simulink model "APFI_MI"  (R2025a)
settings: Solver=VariableStepAuto  StartTime=0.0  StopTime=1  RelTol=1e-3
undefined symbols (not defined in the file): Capacitor, Start
libraries: spsSeriesRLCBranchLib x4, spsBreakerLib x3, spsACVoltageSourceLib x1, spsCurrentMeasurementLib x1, spsPowerLib x1, spsSinglePhaseAsynchronousMachineLib x1, spsVoltageMeasurementLib x1, spspowerguiLib x1
settings Model: PacingRate=0.100000  Creator=saman  LastModifiedBy=shaik
settings SolverCC: ZeroCrossAlgorithm=Adaptive
settings DebuggingCC: IgnoredZcDiagnostic=none  UnconnectedInputMsg=warning  UnconnectedOutputMsg=warning  UnconnectedLineMsg=warning
settings ModelReferenceCC: EnableRefExpFcnMdlSchedulingChecks=on
settings RTWCC: GPUComputeCapability=3.5  DLArmComputeVersion=19.05

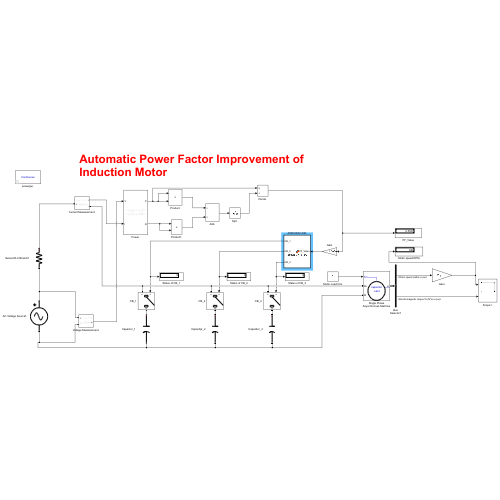
[thumbnail: Simulink's stored preview of the top-level diagram]
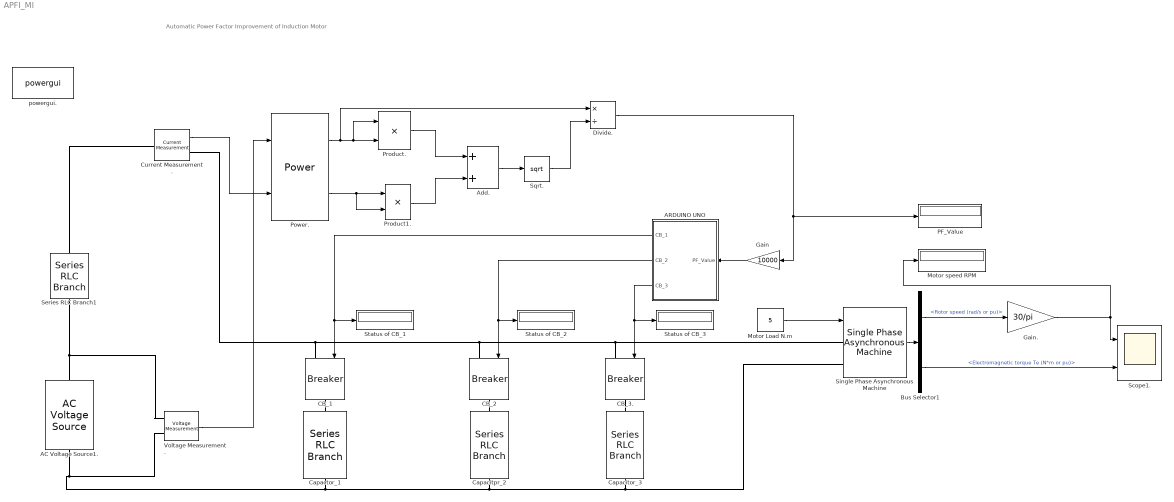
== system APFI_MI ==
  note: Automatic Power Factor Improvement of
      | Induction Motor
  AC Voltage Source1. : spsACVoltageSourceLib/AC Voltage Source  Amplitude=311.1  Phase=0  Frequency=50  SampleTime=0  Measurements=None  BusType=swing  Pref=10e3  Qref=0  Qmin=-inf  Qmax=+inf
  ARDUINO UNO : MATLAB Function  TreatAsAtomicUnit=on  SystemSampleTime=0.9
  Add. : Sum
  Bus Selector1 : BusSelector  OutputSignals=Mechanical.Rotor speed (rad/s or pu),Mechanical.Electromagnetic torque Te (N*m or pu)
  CB_1 : spsBreakerLib/Breaker  InitialState=0  SwitchingTimes="[1/60  5/60]"  External=on  BreakerResistance=0  SnubberResistance=0  SnubberCapacitance=0  Measurements=None  MoreParameters=on  NoBreakLoop=off
  CB_2 : spsBreakerLib/Breaker  InitialState=0  SwitchingTimes="[1/60  5/60]"  External=on  BreakerResistance=0  SnubberResistance=0  SnubberCapacitance=0  Measurements=None  MoreParameters=on  NoBreakLoop=off
  CB_3. : spsBreakerLib/Breaker  InitialState=0  SwitchingTimes="[1/60  5/60]"  External=on  BreakerResistance=0  SnubberResistance=0  SnubberCapacitance=0  Measurements=None  MoreParameters=on  NoBreakLoop=off
  Capacitor_3 : spsSeriesRLCBranchLib/Series RLC Branch  LConnTagsString=__new0  RConnTagsString=__new0  BranchType=C  Resistance=1  Inductance=1e-3  SetiL0=off  InitialCurrent=0  Capacitance=65e-6  Setx0=off  InitialVoltage=0  Measurements=None
  Capacitpr_2 : spsSeriesRLCBranchLib/Series RLC Branch  LConnTagsString=__new0  RConnTagsString=__new0  BranchType=C  Resistance=1  Inductance=1e-3  SetiL0=off  InitialCurrent=0  Capacitance=40e-6  Setx0=off  InitialVoltage=0  Measurements=None
  Capactor_1 : spsSeriesRLCBranchLib/Series RLC Branch  LConnTagsString=__new0  RConnTagsString=__new0  BranchType=C  Resistance=1  Inductance=1e-3  SetiL0=off  InitialCurrent=0  Capacitance=70e-6  Setx0=off  InitialVoltage=0  Measurements=None
  Current Measurement. : spsCurrentMeasurementLib/Current Measurement  PhasorSimulation=off  OutputType=Complex  PSBequivalent=0
  Divide. : Product  Inputs=*/
  Gain : Gain  Gain=10000
  Gain. : Gain  Gain=30/pi
  Motor Load N.m : Constant  Value=5
  Motor speed RPM : Display
  PF_Value : Display
  Power. : spsPowerLib/Power  Freq=50  Vinit=[1, 0]  Iinit=[1, 0]  Ts=0
  Product. : Product
  Product1. : Product
  Scope1. : Scope  NumInputPorts=2
      settings: ActiveDisplayYMinimum=-191.13592  ActiveDisplayYMaximum=1609.96968  DataLoggingVariableName=ScopeData3
  Series RLC Branch1 : spsSeriesRLCBranchLib/Series RLC Branch  LConnTagsString=__new0  RConnTagsString=__new0  BranchType=R  Resistance=2  Inductance=1e-3  SetiL0=off  InitialCurrent=0  Capacitance=1e-6  Setx0=off  InitialVoltage=0  Measurements=None
  Single Phase Asynchronous Machine : spsSinglePhaseAsynchronousMachineLib/Single Phase Asynchronous Machine  MechanicalLoad=Torque Tm  UNITS=SI  MachineType=Capacitor-Start  MeasurementBus=off  NominalParameters="[ .5*746  311  50]"  MainWindingStator="[2.02  25.4e-3]"  MainWindingRotor="[4.12  20.6e-3]"  MutualInductance=0.1773  AuxiliaryWinding="[7.14  8.5e-3]"  Mechanical="[0.014  0  2 1]"  CapacitorStart="[2  254.7e-6]"  CapacitorRun="[18  21.1e-6]"  DisconnectionSpeed=75  InitialSpeed=0  DataType=SI  TsPowergui=0  TsBlock=-1
  Sqrt. : Sqrt
  Status of CB_1 : Display
  Status of CB_2 : Display
  Status of CB_3 : Display
  Voltage Measurement. : spsVoltageMeasurementLib/Voltage Measurement  PhasorSimulation=off  OutputType=Complex  PSBequivalent=0
  powergui. : spspowerguiLib/powergui  Priority=1  SimulationMode=Continuous  SampleTime=50e-6  frequency=60  Iterations=50  frequencyindice=50  Pbase=100e6  ErrMax=1e-4  UnitsV=kV  UnitsW=MW  buscounter=0  FunctionMessages=off  echomessages=off  EnableUseOfTLC=off  CurrentSourceSwitches=off  DisableSnubberDevices=off  DisableRonSwitches=off  DisableVfSwitches=off  DisplayEquations=off  AutomaticDiscreteSolvers=off  SolverType=Tustin/Backward Euler (TBE)  Interpol=off  ExternalGateDelay=off  methode=off  Ts=100  x0status=blocks  SPID=on  SwTol=0  HookPort=off  NonlinearTolerance=1e-4  nMaxIteration=100  ContinueOnMaxIteration=off  RestoreLinks=warning  ResistiveCurrentMeasurement=off  Frange=[0:2:500]  Ylog=off  Xlog=on  ShowGrid=off  save=off  variable=ZData  structure=0  ZoomFFT=off  StartTime=0.0  cycles=1  DisplayStyle=1  fundamental=60  FreqAxis=off  MaxFrequency=1000  frequencyindicesteady=1  RmsSteady=1  display=off
  wires:
  Product./1 -> Add./1
  Current Measurement./1 -> Power./2
  Bus Selector1/2 -> Scope1./2  "<Electromagnetic torque Te (N*m or pu)>"
  Divide./1 -> Gain/1, PF_Value/1
  Gain./1 -> Scope1./1, Motor speed RPM/1
  Sqrt./1 -> Divide./2
  Voltage Measurement./1 -> Power./1
  Power./1 -> Divide./1, Product./1, Product./2
  Single Phase Asynchronous Machine/1 -> Bus Selector1/1
  Motor Load N.m/1 -> Single Phase Asynchronous Machine/1
  Product1./1 -> Add./2
  Add./1 -> Sqrt./1
  Bus Selector1/1 -> Gain./1  "<Rotor speed (rad/s or pu)>"
  Power./2 -> Product1./2, Product1./1
  ARDUINO UNO/1(CB_1) -> CB_1/1, Status of CB_1/1
  ARDUINO UNO/2(CB_2) -> Status of CB_2/1, CB_2/1
  ARDUINO UNO/3(CB_3) -> CB_3./1, Status of CB_3/1
  Gain/1 -> ARDUINO UNO/1(PF_Value)
  connections:
  AC Voltage Source1./RConn1 -- Series RLC Branch1/RConn1 -- Voltage Measurement./LConn1
  Capacitpr_2/LConn1 -- CB_2/RConn1
  CB_3./RConn1 -- Capacitor_3/LConn1
  Series RLC Branch1/LConn1 -- Current Measurement./LConn1
  Current Measurement./RConn1 -- CB_2/LConn1 -- Single Phase Asynchronous Machine/LConn1 -- CB_3./LConn1 -- CB_1/LConn1
  AC Voltage Source1./LConn1 -- Single Phase Asynchronous Machine/LConn2 -- Capacitor_3/RConn1 -- Capacitpr_2/RConn1 -- Capactor_1/RConn1 -- Voltage Measurement./LConn2
  Capactor_1/LConn1 -- CB_1/RConn1

== matlab function APFI_MI/ARDUINO UNO ==
  data: CB_1 output; CB_2 output; PF_Value input; CB_3 output
function [CB_1,CB_2,CB_3] = ARDUINO_UNO(PF_Value)
   
  
        if PF_Value>4999 && PF_Value<5002
                CB_1=1;
                CB_2=0;
                CB_3=0;
                return
        end
        if PF_Value>5862 && PF_Value<5866
                CB_1=1;
                CB_2=1;
                CB_3=0;
                return
        end
        if PF_Value>5245 && PF_Value<5249
                CB_1=1;
                CB_2=1;
                CB_3=1;
                return
        else
                CB_1=0;
                CB_2=0;
                CB_3=0;
        end
end
